simulink model "TaskC"  (R2022b)
settings: Solver=ode45  StartTime=0.0  StopTime=10.0  RelTol=1e-3
undefined symbols (not defined in the file): A_aug_sine, absolute_encoder_counts_per_revolution, B_aug_sine, C_aug_sine, Cd_sine, DiscIntNeverNeededParam, init, K_I2, K_x2, Lsine, w
libraries: simulink_extras x6
settings Model: Creator=tumisangramotlhwa  LastModifiedBy=tumisangramotlhwa

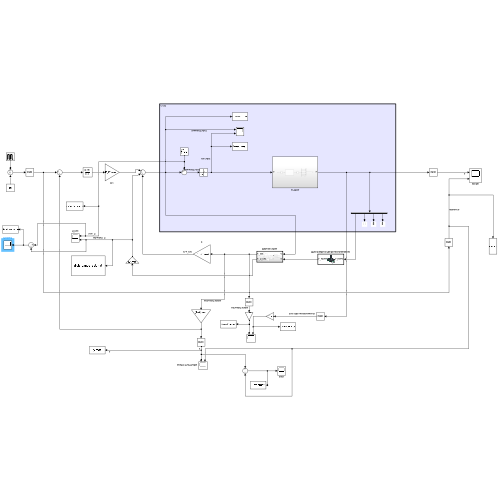
[thumbnail: Simulink's stored preview of the top-level diagram]
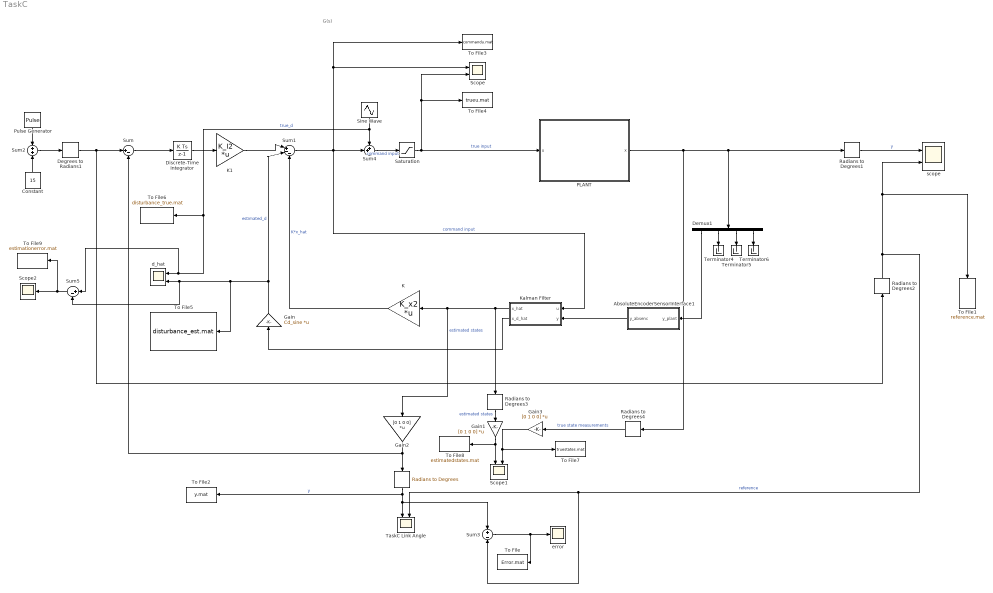
== system TaskC ==
  note: G(s)
  " " : simulink_extras/Transformations/Radians to Degrees
  AbsoluteEncoderSensorInterface1 : Subsystem  TreatAsAtomicUnit=on
      mask Display: image('$imagefile'); % Use "Edit Image" on toolstrip to change.
  Constant : Constant  Value=15
  Degrees to Radians1 : simulink_extras/Transformations/Degrees to Radians
  Demux1 : Demux
  Discrete-Time Integrator : DiscreteIntegrator  SampleTime=-1  ICPrevOutput=DiscIntNeverNeededParam  ICPrevScaledInput=DiscIntNeverNeededParam
  Gain : Gain  Gain=Cd_sine  Multiplication=Matrix(K*u) (u vector)
  Gain1 : Gain  Gain=[0 1 0 0]  Multiplication=Matrix(K*u) (u vector)
  Gain2 : Gain  Gain=[0 1 0 0]  Multiplication=Matrix(K*u) (u vector)
  Gain3 : Gain  Gain=[0 1 0 0]  Multiplication=Matrix(K*u) (u vector)
  K : Gain  Gain=K_x2  Multiplication=Matrix(K*u) (u vector)
  K1 : Gain  Gain=K_I2  Multiplication=Matrix(K*u) (u vector)
  Kalman Filter : Subsystem  TreatAsAtomicUnit=on
  PLANT : Subsystem
  Pulse Generator : DiscretePulseGenerator  PulseType=Time based  Amplitude=30  Period=4  PulseWidth=50
  Radians to Degrees{1..4} (4 alike) : simulink_extras/Transformations/Radians to Degrees
  Saturation : Saturate  UpperLimit=6  LowerLimit=-6
  Scope : Scope  NumInputPorts=2
  Scope1 : Scope  NumInputPorts=2
  Scope2 : Scope
  Sine Wave : Sin  Amplitude=0.3  Frequency=w  SampleTime=0
  Sum : Sum  Inputs=|+-
  Sum1 : Sum  Inputs=|+--
  Sum2 : Sum  Inputs=+|+
  Sum3 : Sum  Inputs=+|-
  Sum4 : Sum  Inputs=++|
  Sum5 : Sum  Inputs=|+-
  TaskC Link Angle : Scope  NumInputPorts=2
  Terminator4 : Terminator
  Terminator5 : Terminator
  Terminator6 : Terminator
  To File : ToFile  Filename=Error.mat  MatrixName=Error  SaveFormat=Timeseries
  To File1 : ToFile  Filename=reference.mat  MatrixName=reference  SaveFormat=Timeseries
  To File2 : ToFile  Filename=y.mat  MatrixName=y  SaveFormat=Timeseries
  To File3 : ToFile  Filename=commandu.mat  MatrixName=commandu  SaveFormat=Timeseries
  To File4 : ToFile  Filename=trueu.mat  MatrixName=trueu  SaveFormat=Timeseries
  To File5 : ToFile  Filename=disturbance_est.mat  MatrixName=disturbance_est  SaveFormat=Timeseries
  To File6 : ToFile  Filename=disturbance_true.mat  MatrixName=disturbance_true  SaveFormat=Timeseries
  To File7 : ToFile  Filename=truestates.mat  MatrixName=truestates  SaveFormat=Timeseries
  To File8 : ToFile  Filename=estimatedstates.mat  MatrixName=estimatedstates  SaveFormat=Timeseries
  To File9 : ToFile  Filename=estimationerror.mat  MatrixName=estimationerror  SaveFormat=Timeseries
  d_hat : Scope  NumInputPorts=2
  error : Scope
  scope : Scope  NumInputPorts=2
  wires:
  Sum2/1 -> Degrees to Radians1/1
  K1/1 -> Sum1/1
  Constant/1 -> Sum2/2
  Radians to Degrees2/1 -> Sum3/2, TaskC Link Angle/2, scope/2, To File1/1  "reference"
  Degrees to Radians1/1 -> Radians to Degrees2/1, Sum/1
  Radians to Degrees4/1 -> Gain3/1  "true state measurements"
  Demux1/2 -> Terminator4/1
  Radians to Degrees1/1 -> scope/1  "y"
  Demux1/3 -> Terminator5/1
  Radians to Degrees3/1 -> Gain1/1  "estimated states"
  Demux1/1 -> AbsoluteEncoderSensorInterface1/1(y_plant)
  Pulse Generator/1 -> Sum2/1
  PLANT/1(x) -> Radians to Degrees1/1, Demux1/1, Radians to Degrees4/1
  Saturation/1 -> PLANT/1(u), To File4/1, Scope/2  "true input"
  K/1 -> Sum1/3  "K*x_hat"
  Demux1/4 -> Terminator6/1
  Gain2/1 -> Sum/2, " "/1
  Kalman Filter/1(x_hat) -> Gain2/1, K/1, Radians to Degrees3/1  "estimated states"
  Discrete-Time Integrator/1 -> K1/1
  Kalman Filter/2(x_d_hat) -> Gain/1
  Gain/1 -> Sum1/2, To File5/1, d_hat/2, Sum5/2  "estimated_d"
  Sine Wave/1 -> To File6/1, Sum5/1, d_hat/1, Sum4/1  "true_d"
  Sum4/1 -> Saturation/1  "command input"
  Sum/1 -> Discrete-Time Integrator/1
  Sum3/1 -> To File/1, error/1
  AbsoluteEncoderSensorInterface1/1(y_absenc) -> Kalman Filter/2(y)
  Sum1/1 -> Kalman Filter/1(u), Scope/1, To File3/1, Sum4/2  "command input"
  " "/1 -> TaskC Link Angle/1, Sum3/1, To File2/1  "y"
  Gain1/1 -> To File8/1, Scope1/1
  Gain3/1 -> Scope1/2, To File7/1
  Sum5/1 -> Scope2/1, To File9/1

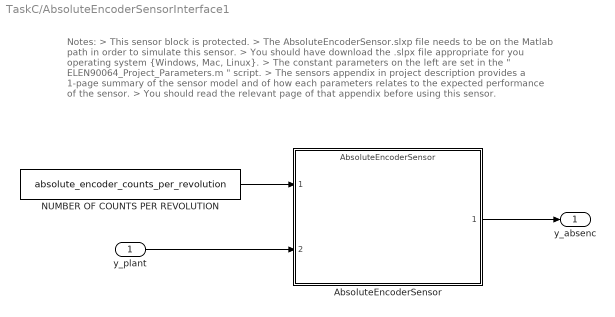
== system TaskC/AbsoluteEncoderSensorInterface1 ==
  note: Notes:
      | > This sensor block is protected.
      | > The AbsoluteEncoderSensor.slxp file needs to be on the Matlab path in order to simulate this sensor.
      | > You should have download the .slpx file appropriate for you operating system {Windows, Mac, Linux}.
      | > The constant parameters on the left are set in the " ELEN90064_Project_Parameters.m " script.
      | > The sensors appendix in project description provides a 1-page summary of the sensor model and of how each parameters relates to the expected performance of the sensor.
      | > You should read the relevant page of that appendix before using this sensor.
  y_plant : Inport
  AbsoluteEncoderSensor : ModelReference  ModelNameDialog=AbsoluteEncoderSensor.slxp  ModelReferenceVersion=1.16  CopyOfModelProtected=on
  NUMBER OF COUNTS PER REVOLUTION : Constant  Value=absolute_encoder_counts_per_revolution
  y_absenc : Outport
  wires:
  NUMBER OF COUNTS PER REVOLUTION/1 -> AbsoluteEncoderSensor/1
  y_plant/1 -> AbsoluteEncoderSensor/2
  AbsoluteEncoderSensor/1 -> y_absenc/1

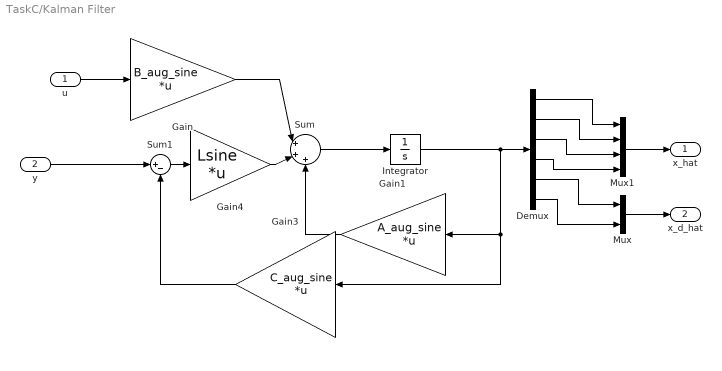
== system TaskC/Kalman Filter ==
  u : Inport
  y : Inport  Port=2
  Demux : Demux  Outputs=6
  Gain : Gain  Gain=B_aug_sine  Multiplication=Matrix(K*u) (u vector)
  Gain1 : Gain  Gain=A_aug_sine  Multiplication=Matrix(K*u) (u vector)
  Gain3 : Gain  Gain=C_aug_sine  Multiplication=Matrix(K*u) (u vector)
  Gain4 : Gain  Gain=Lsine  Multiplication=Matrix(K*u) (u vector)
  Integrator : Integrator
  Mux : Mux  Inputs=2
  Mux1 : Mux
  Sum : Sum  Inputs=|+++
  Sum1 : Sum  Inputs=|+-
  x_hat : Outport
  x_d_hat : Outport  Port=2
  wires:
  Gain/1 -> Sum/1
  Gain4/1 -> Sum/2
  Sum1/1 -> Gain4/1
  Gain3/1 -> Sum1/2
  Gain1/1 -> Sum/3
  Sum/1 -> Integrator/1
  Integrator/1 -> Gain1/1, Gain3/1, Demux/1
  u/1 -> Gain/1
  y/1 -> Sum1/1
  Mux1/1 -> x_hat/1
  Demux/1 -> Mux1/1
  Demux/2 -> Mux1/2
  Demux/3 -> Mux1/3
  Demux/4 -> Mux1/4
  Mux/1 -> x_d_hat/1
  Demux/5 -> Mux/1
  Demux/6 -> Mux/2

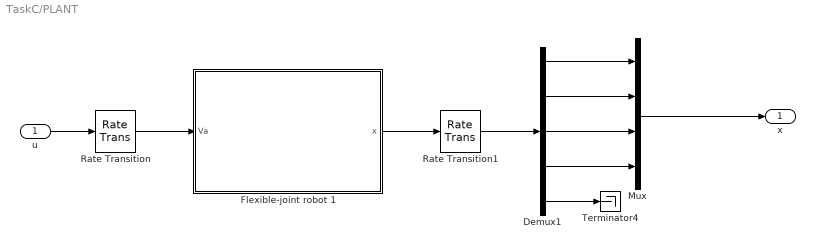
== system TaskC/PLANT ==
  u : Inport
  Demux1 : Demux  Outputs=5
  Flexible-joint robot 1 : Subsystem
      mask Display: image('$imagefile'); % Use "Edit Image" on toolstrip to change.
  Mux : Mux
  Rate Transition : RateTransition  OutPortSampleTime=Ts
  Rate Transition1 : RateTransition  OutPortSampleTime=Ts
  Terminator4 : Terminator
  x : Outport
  wires:
  Demux1/4 -> Mux/4
  Demux1/3 -> Mux/3
  Demux1/2 -> Mux/2
  Demux1/1 -> Mux/1
  Demux1/5 -> Terminator4/1
  u/1 -> Rate Transition/1
  Mux/1 -> x/1
  Flexible-joint robot 1/1(x) -> Rate Transition1/1
  Rate Transition1/1 -> Demux1/1
  Rate Transition/1 -> Flexible-joint robot 1/1(Va)

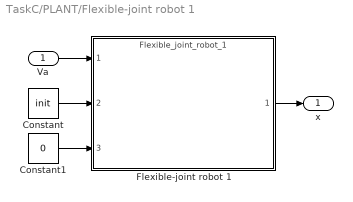
== system TaskC/PLANT/Flexible-joint robot 1 ==
  Va : Inport
  Constant : Constant  Value=init
  Constant1 : Constant  Value=0
  Flexible-joint robot 1 : ModelReference  ModelNameDialog=Flexible_joint_robot_1  ModelReferenceVersion=1.63  CopyOfModelProtected=on
  x : Outport
  wires:
  Constant/1 -> Flexible-joint robot 1/2
  Constant1/1 -> Flexible-joint robot 1/3
  Flexible-joint robot 1/1 -> x/1
  Va/1 -> Flexible-joint robot 1/1
